simulink subsystem "publisher"  (R2021a)
settings: Solver=VariableStepAuto  StartTime=0.0  StopTime=10.0  RelTol=1e-3
values from neighbouring files (symbols this model uses):
  L = 0.32    [ros_cacc.m]    (also in ros_cacc2.m)
  v_0 = 0.5    [ros_cacc.m]    (also in ros_cacc2.m)
  v_threshold = v_thr    (= 0.1)    [ros_cacc.m]    (also in ros_cacc2.m)
undefined symbols (not defined in the file or in its folder): angular, linear
libraries: ros2lib x4, robotcorelib x1
settings Model: Creator=harun  LastModifiedBy=harun

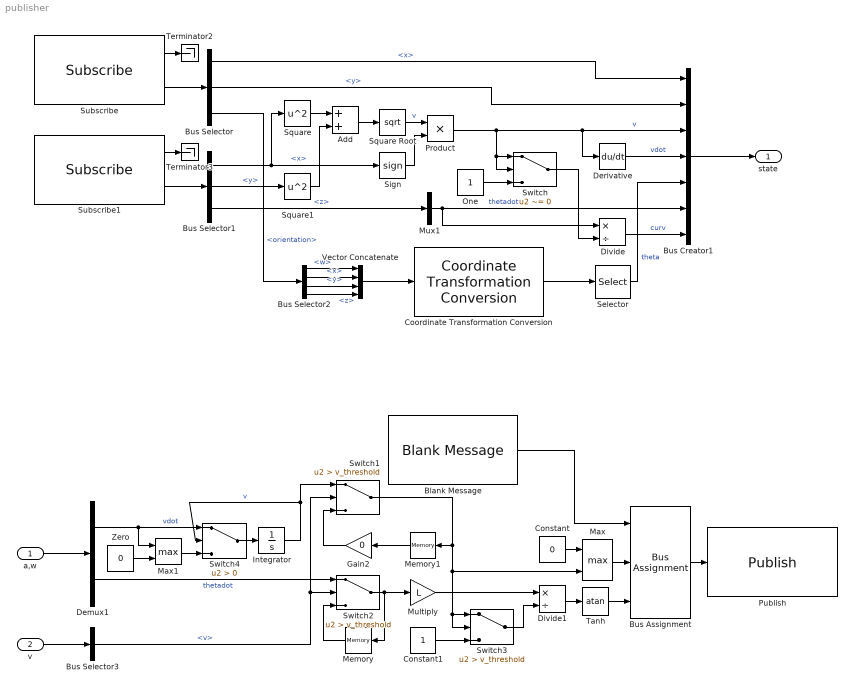
== system publisher ==
  a,w : Inport
  v : Inport  Port=2
  Add : Sum
  Blank Message : ros2lib/Blank Message  messageType=geometry_msgs/Twist  SampleTime=0.01
      settings: SourceProductBaseCode=RR
  Bus Assignment : BusAssignment  AssignedSignals=linear.x,angular.z
  Bus Creator1 : BusCreator  Inputs=7
  Bus Selector : BusSelector  OutputSignals=pose.position.x,pose.position.y,pose.orientation
  Bus Selector1 : BusSelector  OutputSignals=twist.twist.linear.x,twist.twist.linear.y,twist.twist.angular.z
  Bus Selector2 : BusSelector  OutputSignals=w,x,y,z
  Bus Selector3 : BusSelector  OutputSignals=v
  Constant : Constant  Value=0
  Constant1 : Constant
  Coordinate Transformation Conversion : robotcorelib/Coordinate Transformation Conversion  InputRepresentation=Quaternion  InputEulerSequence=ZYX  ShowTrVecInputPort=on  OutputRepresentation=Euler Angles  OutputEulerSequence=ZYX  ShowTrVecOutputPort=on  SimulateUsing=Interpreted execution
      settings: SourceProductBaseCode=NV,RO,RR,UV
  Demux1 : Demux  Outputs=2
  Derivative : Derivative
  Divide : Product  Inputs=*/
  Divide1 : Product  Inputs=*/
  Gain2 : Gain  Gain=0
  Integrator : Integrator  InitialCondition=v_0
  Max : MinMax  Function=max  Inputs=2
  Max1 : MinMax  Function=max  Inputs=2
  Memory : Memory
  Memory1 : Memory
  Multiply : Gain  Gain=L
  Mux1 : Mux  Inputs=1
  One : Constant  OutDataTypeStr=Inherit: Inherit via back propagation
  Product : Product
  Publish : ros2lib/Publish  topicSource=Specify your own  topic=/robot3/cmd_vel  messageType=geometry_msgs/Twist  QOSHistory=Keep last  QOSDepth=1  QOSReliability=Reliable  QOSDurability=Volatile
      settings: SourceProductBaseCode=RR
  Selector : Selector  InputPortWidth=3  IndexOptions=Index vector (dialog)  Indices=[1]  OutputSizes=1
  Sign : Signum
  Square : Math  Operator=square  SaturateOnIntegerOverflow=on
  Square Root : Sqrt  SaturateOnIntegerOverflow=on
  Square1 : Math  Operator=square  SaturateOnIntegerOverflow=on
  Subscribe : ros2lib/Subscribe  topicSource=Specify your own  topic=/robot3/robot_pose  messageType=geometry_msgs/PoseStamped  sampleTime=0.01  QOSHistory=Keep last  QOSDepth=1  QOSReliability=Reliable  QOSDurability=Volatile
      settings: SourceProductBaseCode=RR
  Subscribe1 : ros2lib/Subscribe  topicSource=Specify your own  topic=/robot3/odom  messageType=nav_msgs/Odometry  sampleTime=0.01  QOSHistory=Keep last  QOSDepth=1  QOSReliability=Reliable  QOSDurability=Volatile
      settings: SourceProductBaseCode=RR
  Switch : Switch  Criteria=u2 ~= 0
  Switch1 : Switch  Criteria=u2 > Threshold  Threshold=v_threshold
  Switch2 : Switch  Criteria=u2 > Threshold  Threshold=v_threshold
  Switch3 : Switch  Criteria=u2 > Threshold  Threshold=v_threshold
  Switch4 : Switch  Criteria=u2 > Threshold
  Tanh : Trigonometry  Operator=atan
  Terminator2 : Terminator
  Terminator3 : Terminator
  Vector Concatenate : Concatenate  NumInputs=4
  Zero : Constant  Value=0  OutDataTypeStr=Inherit: Inherit via back propagation
  state : Outport  VectorParamsAs1DForOutWhenUnconnected=off
  wires:
  Bus Selector2/3 -> Vector Concatenate/3  "<y>"
  Subscribe1/1 -> Terminator3/1
  Demux1/2 -> Switch2/1  "thetadot"
  Memory1/1 -> Gain2/1
  Max/1 -> Bus Assignment/2
  One/1 -> Switch/3
  Bus Selector1/3 -> Mux1/1  "<z>"
  Vector Concatenate/1 -> Coordinate Transformation Conversion/1
  Bus Selector1/2 -> Square1/1  "<y>"
  Divide1/1 -> Tanh/1
  Bus Selector2/2 -> Vector Concatenate/2  "<x>"
  Bus Selector/3 -> Bus Selector2/1  "<orientation>"
  v/1 -> Bus Selector3/1
  Subscribe/1 -> Terminator2/1
  Bus Selector1/1 -> Sign/1, Square/1  "<x>"
  Bus Selector/1 -> Bus Creator1/1  "<x>"
  Mux1/1 -> Bus Creator1/6, Divide/1  "thetadot"
  Add/1 -> Square Root/1
  Bus Selector/2 -> Bus Creator1/2  "<y>"
  Bus Selector2/4 -> Vector Concatenate/4  "<z>"
  Selector/1 -> Bus Creator1/5  "theta"
  Square/1 -> Add/1
  Memory/1 -> Switch2/3
  Integrator/1 -> Switch4/2, Switch1/1  "v"
  Bus Creator1/1 -> state/1
  Square Root/1 -> Product/1  "v"
  Switch2/1 -> Memory/1, Multiply/1
  Sign/1 -> Product/2
  Coordinate Transformation Conversion/1 -> Selector/1
  Product/1 -> Bus Creator1/3, Derivative/1, Switch/2, Switch/1  "v"
  a,w/1 -> Demux1/1
  Switch4/1 -> Integrator/1
  Constant/1 -> Max/1
  Multiply/1 -> Divide1/1
  Bus Selector2/1 -> Vector Concatenate/1  "<w>"
  Subscribe1/2 -> Bus Selector1/1
  Blank Message/1 -> Bus Assignment/1
  Switch3/1 -> Divide1/2
  Divide/1 -> Bus Creator1/7  "curv"
  Square1/1 -> Add/2
  Constant1/1 -> Switch3/3
  Tanh/1 -> Bus Assignment/3
  Switch1/1 -> Memory1/1, Switch3/2, Switch3/1, Max/2
  Gain2/1 -> Switch1/3
  Demux1/1 -> Switch4/1, Max1/1  "vdot"
  Bus Assignment/1 -> Publish/1
  Derivative/1 -> Bus Creator1/4  "vdot"
  Subscribe/2 -> Bus Selector/1
  Zero/1 -> Max1/2
  Bus Selector3/1 -> Switch1/2, Switch2/2  "<v>"
  Max1/1 -> Switch4/3
  Switch/1 -> Divide/2
